simulink model "Question_2_Lead_Compensator"  (Simulink 10.3)
settings: Solver=VariableStepAuto  StartTime=0.0  StopTime=2  RelTol=1e-3
libraries: simulink x2
settings Model: Creator=Electrical Dept  LastModifiedBy=mofid  MultithreadedSim=on
settings DataIOCC: SaveFormat=Dataset  SignalLoggingSaveFormat=Dataset  ReturnWorkspaceOutputs=on
settings OptimizationCC: ExpressionDepthLimit=128  LifeSpan=auto
settings DebuggingCC: UnderspecifiedInitializationDetection=Simplified  MergeDetectMultiDrivingBlocksExec=error  FcnCallInpInsideContextMsg=error  StateNameClashWarn=none  SFUnexpectedBacktrackingDiag=error  SFNoUnconditionalDefaultTransitionDiag=error  SFExecutionAtInitializationDiag=warning  ArithmeticOperatorsInVariantConditions=error
settings HardwareCC: ProdBitPerPointer=64  ProdBitPerSizeT=64  ProdBitPerPtrDiffT=64  ProdLargestAtomicFloat=Float  ProdIntDivRoundTo=Zero  ProdEndianess=LittleEndian  ProdWordSize=64  ProdHWDeviceType=Intel->x86-64 (Windows64)
settings ModelReferenceCC: PropagateSignalLabelsOutOfModel=on
settings SFSimCC: SimUseLocalCustomCode=on
settings RTWCC: RTWUseLocalCustomCode=on  DLArmComputeVersion=20.02.1
settings CodeAppCC: StateflowObjectComments=off
settings GRTTargetCC: TargetLangStandard=C99 (ISO)  CombineOutputUpdateFcns=on  GRTInterface=off
settings ConfigComp: CovMetricSettings=dwe  CovSaveCumulativeToWorkspaceVar=off  CovSaveSingleToWorkspaceVar=off  CovExternalEMLEnable=on

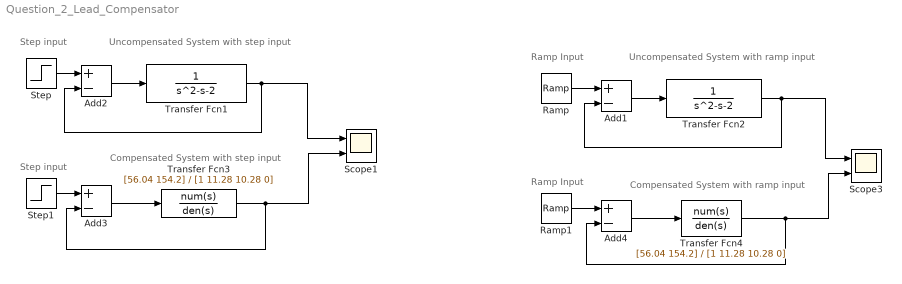
== system Question_2_Lead_Compensator ==
  note: Ramp Input
  note: Step input
  note: Compensated System with step input
  note: Uncompensated System with step input
  note: Compensated System with ramp input
  note: Uncompensated System with ramp input
  note: Step input
  note: Ramp Input
  Add{1..4} (4 alike) : Sum  Inputs=+-
  Ramp : simulink/Sources/Ramp  slope=1  start=0  InitialOutput=0
  Ramp1 : simulink/Sources/Ramp  slope=1  start=0  InitialOutput=0
  Scope1 : Scope  NumInputPorts=2
  Scope3 : Scope  NumInputPorts=2
  Step : Step  Time=0  SampleTime=0
  Step1 : Step  Time=0  SampleTime=0
  Transfer Fcn1 : TransferFcn  Denominator=[1 -1 -2]
  Transfer Fcn2 : TransferFcn  Denominator=[1 -1 -2]
  Transfer Fcn3 : TransferFcn  Numerator=[56.04 154.2]  Denominator=[1 11.28 10.28 0]
  Transfer Fcn4 : TransferFcn  Numerator=[56.04 154.2]  Denominator=[1 11.28 10.28 0]
  wires:
  Add2/1 -> Transfer Fcn1/1
  Transfer Fcn1/1 -> Add2/2, Scope1/1
  Transfer Fcn3/1 -> Scope1/2, Add3/2
  Add3/1 -> Transfer Fcn3/1
  Step/1 -> Add2/1
  Step1/1 -> Add3/1
  Ramp1/1 -> Add4/1
  Ramp/1 -> Add1/1
  Add4/1 -> Transfer Fcn4/1
  Transfer Fcn4/1 -> Add4/2, Scope3/2
  Transfer Fcn2/1 -> Add1/2, Scope3/1
  Add1/1 -> Transfer Fcn2/1
